simulink model "Q_3"  (R2020a)
settings: Solver=VariableStepAuto  StartTime=0.0  StopTime=10.0  RelTol=1e-3
settings Model: Creator=Admin  LastModifiedBy=Admin

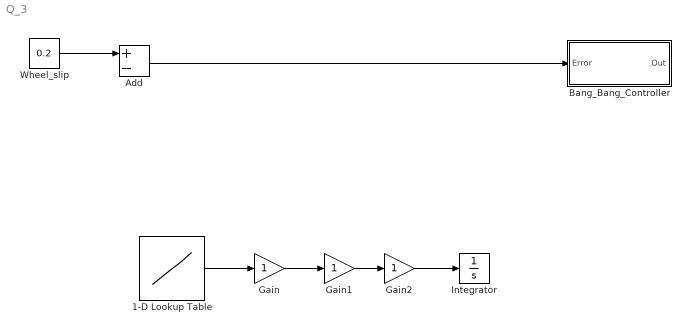
== system Q_3 ==
  1-D Lookup Table : Lookup_n-D  NumberOfTableDimensions=1  BreakpointsForDimension1=[-5:5]  Table=tanh([-5:5])  InternalRulePriority=Speed  RndMeth=Simplest  InputSameDT=on
  Add : Sum  Inputs=+-
  Bang_Bang_Controller : Subsystem  TreatAsAtomicUnit=on
  Gain : Gain
  Gain1 : Gain
  Gain2 : Gain
  Integrator : Integrator
  Wheel_slip : Constant  Value=0.2
  wires:
  Wheel_slip/1 -> Add/1
  ? -> Add/2
  Gain/1 -> Gain1/1
  Gain1/1 -> Gain2/1
  Gain2/1 -> Integrator/1
  1-D Lookup Table/1 -> Gain/1
  Add/1 -> Bang_Bang_Controller/1(Error)

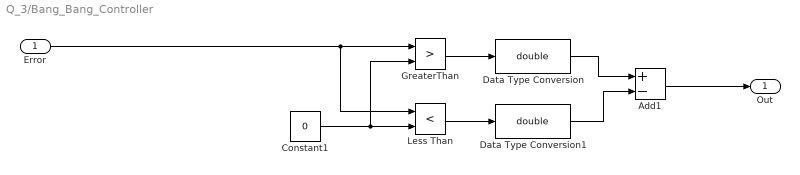
== system Q_3/Bang_Bang_Controller ==
  Error : Inport
  Add1 : Sum  Inputs=+-
  Constant1 : Constant  Value=0
  Data Type Conversion : DataTypeConversion  OutDataTypeStr=double
  Data Type Conversion1 : DataTypeConversion  OutDataTypeStr=double
  GreaterThan : RelationalOperator  Operator=>  OutDataTypeStr=boolean  RndMeth=Simplest
  Less Than : RelationalOperator  Operator=<  OutDataTypeStr=boolean  RndMeth=Simplest
  Out : Outport
  wires:
  Data Type Conversion1/1 -> Add1/2
  Error/1 -> Less Than/1, GreaterThan/1
  GreaterThan/1 -> Data Type Conversion/1
  Data Type Conversion/1 -> Add1/1
  Add1/1 -> Out/1
  Less Than/1 -> Data Type Conversion1/1
  Constant1/1 -> GreaterThan/2, Less Than/2
